simulink model "trialsGASimulink"  (R2017a)
settings: Solver=VariableStepAuto  StartTime=0.0  StopTime=10.0  RelTol=1e-3
settings Model: Creator=Felipe  LastModifiedBy=Felipe

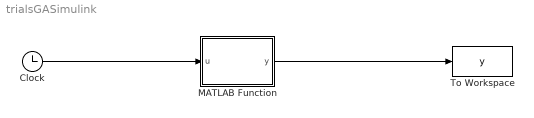
== system trialsGASimulink ==
  Clock : Clock
  MATLAB Function : MATLAB Function  TreatAsAtomicUnit=on
  To Workspace : ToWorkspace  VariableName=y  SaveFormat=Timeseries  SampleTime=-1
  wires:
  Clock/1 -> MATLAB Function/1(u)
  MATLAB Function/1(y) -> To Workspace/1

== matlab function trialsGASimulink/MATLAB Function ==
  data: u input; y output
function y = fcn(u)
% coder.extrinsic('ga');
% coder.extrinsic('optimoptions');
% options =
% optimoptions('ga','UseVectorized',true,'Display','off','MaxStallGenerations',500,'PopulationSize',100,'MaxGenerations',100);
y = 0;
coder.extrinsic('myDummyAssFunction');
y = myDummyAssFunction();
y = y+u(1);
